simulink model "ITMBS_square_M2"  (R2023a)
settings: Solver=FixedStepDiscrete  StartTime=0.0  StopTime=10.0  FixedStep=0.05  RelTol=1e-3  EnableMultiTasking=on
values from neighbouring files (symbols this model uses):
  dist = 100    [M2_square.m]
libraries: legoev3lib x4
settings Model: ExtModeTrigDuration=2  Creator=3w09  LastModifiedBy=Sachin K S
settings SolverCC: PositivePriorityOrder=on  AutoInsertRateTranBlk=on
settings OptimizationCC: EnhancedBackFolding=on  PassReuseOutputArgsAs=Individual arguments  ZeroExternalMemoryAtStartup=off  ZeroInternalMemoryAtStartup=off  MaxStackSize=64  OptimizeBlockOrder=speed  DifferentSizesBufferReuse=on  OptimizationCustomize=off  EfficientTunableParamExpr=on
settings DebuggingCC: ParameterTunabilityLossMsg=error
settings HardwareCC: ProdBitPerPointer=32  ProdBitPerSizeT=32  ProdBitPerPtrDiffT=32  ProdLargestAtomicInteger=Long  ProdWordSize=32  ProdHWDeviceType=ARM Compatible->ARM 9  UseEmbeddedCoderFeatures=off  UseSimulinkCoderFeatures=off
settings SFSimCC: MATLABDynamicMemAlloc=off
settings RTWCC: Description=Embedded Coder  SystemTargetFile=ert.tlc  HardwareBoard=LEGO MINDSTORMS EV3  TLCOptions="-aInlineSetEventsForThisBaseRateFcn=TLC_FALSE -aSuppressMultiTaskScheduler=TLC_FALSE  -aRateBasedStepFcn=0"  TemplateMakefile=ert_default_tmf  Toolchain=Sourcery G++ Lite v2009q3
settings CodeAppCC: ForceParamTrailComments=on  IgnoreCustomStorageClasses=off  OperatorAnnotations=on  SimulinkDataObjDesc=on  SFDataObjDesc=on  InsertBlockDesc=on
settings ERTTargetCC: SupportContinuousTime=on  SupportNonInlinedSFcns=on  SupportVariableSizeSignals=on  ExtModeTransport=2  ExtModeStaticAlloc=on  ExtModeMexFile=ext_xcp  ExtModeIntrfLevel=Level2 - Open

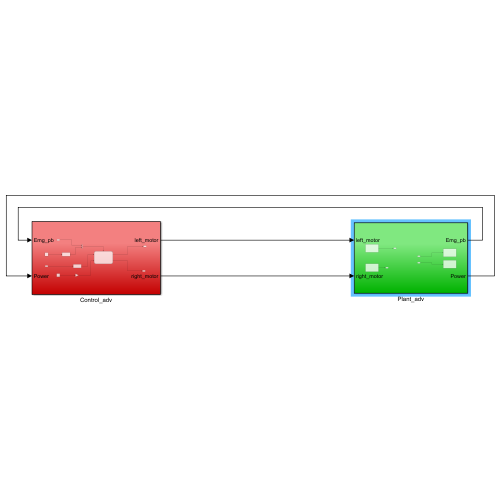
[thumbnail: Simulink's stored preview of the top-level diagram]
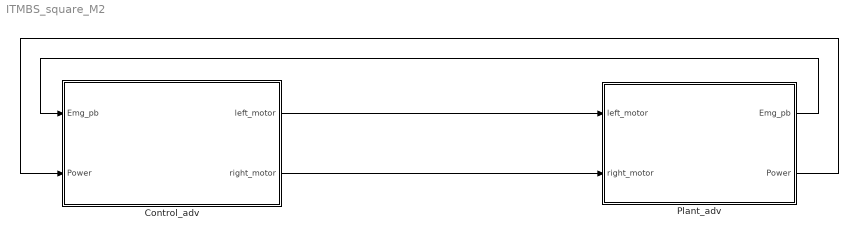
== system ITMBS_square_M2 ==
  Control_adv : Subsystem
  Plant_adv : Subsystem
  wires:
  Plant_adv/1(Emg_pb) -> Control_adv/1(Emg_pb)
  Plant_adv/2(Power) -> Control_adv/2(Power)
  Control_adv/1(left_motor) -> Plant_adv/1(left_motor)
  Control_adv/2(right_motor) -> Plant_adv/2(right_motor)

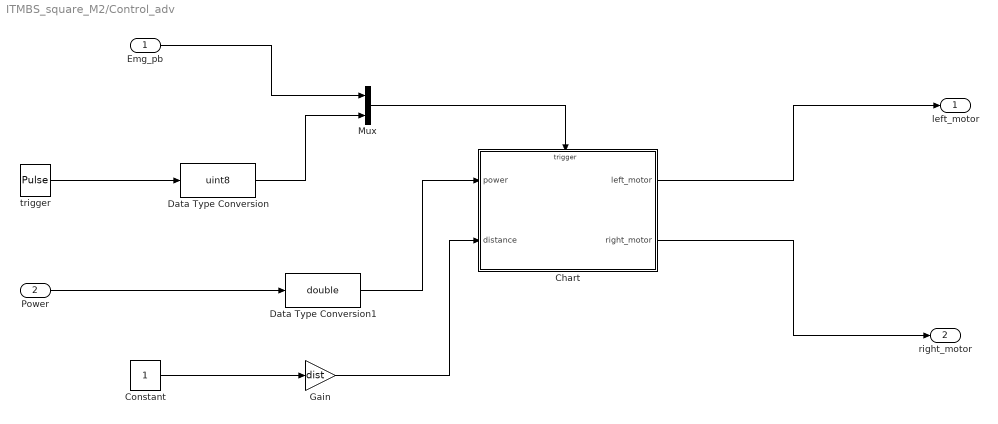
== system ITMBS_square_M2/Control_adv ==
  Emg_pb : Inport
  Power : Inport  Port=2
  Chart : Stateflow chart  TreatAsAtomicUnit=on
  Constant : Constant
  Data Type Conversion : DataTypeConversion  OutDataTypeStr=uint8  SaturateOnIntegerOverflow=off  RndMeth=Floor
  Data Type Conversion1 : DataTypeConversion  OutDataTypeStr=double  SaturateOnIntegerOverflow=off  RndMeth=Floor
  Gain : Gain  Gain=dist
  Mux : Mux  Inputs=2
  trigger : DiscretePulseGenerator  Period=3  PulseWidth=2  SampleTime=0.05
  left_motor : Outport
  right_motor : Outport  Port=2
  wires:
  Constant/1 -> Gain/1
  Emg_pb/1 -> Mux/1
  Chart/2(right_motor) -> right_motor/1
  Gain/1 -> Chart/2(distance)
  Data Type Conversion/1 -> Mux/2
  trigger/1 -> Data Type Conversion/1
  Power/1 -> Data Type Conversion1/1
  Data Type Conversion1/1 -> Chart/1(power)
  Mux/1 -> Chart/Trigger
  Chart/1(left_motor) -> left_motor/1

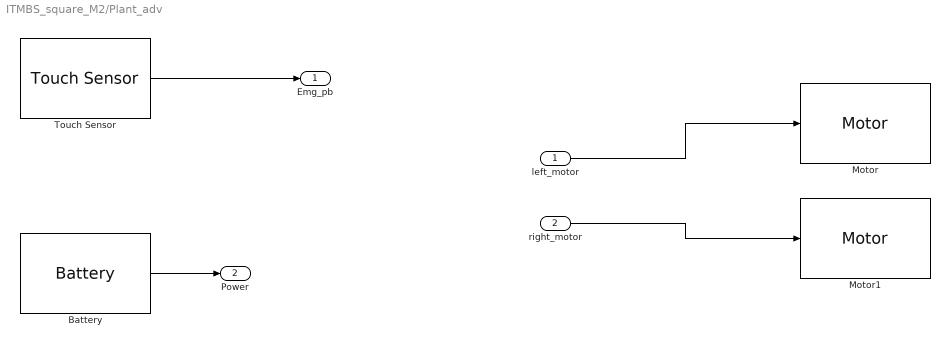
== system ITMBS_square_M2/Plant_adv ==
  left_motor : Inport
  right_motor : Inport  Port=2
  Battery : legoev3lib/Battery  SampleTime=0.1
  Motor : legoev3lib/Motor  sportNumber=A  sstopAction=Brake
  Motor1 : legoev3lib/Motor  sportNumber=B  sstopAction=Brake
  Touch Sensor : legoev3lib/Touch Sensor  portNumber=1  sampleTime=0.1
  Emg_pb : Outport
  Power : Outport  Port=2
  wires:
  Battery/1 -> Power/1
  right_motor/1 -> Motor1/1
  Touch Sensor/1 -> Emg_pb/1
  left_motor/1 -> Motor/1

== stateflow chart ITMBS_square_M2/Control_adv/Chart ==
  settings: executeAtInitialization=1
  state OFF
    entry:
    right_motor=0;
    left_motor=0;
    c=0;
  state ON
    right_motor =power;
    left_motor =power;
  state square
    entry:
    right_motor= 0;
    left_motor=power;
  (default) -> ON
  ON -> OFF [order 1] : [pushbutton_event_input]
  square -> ON [order 2] : [after(0.32,sec)]
  OFF -> (junction 36)
  square -> OFF [order 1] : [pushbutton_event_input]
  ON -> square [order 2] : [after(0.0192* distance ,sec)]
  (junction 38) -> ON [order 1] : [c==2]
  (junction 36) -> (junction 37) [order 1] : [pushbutton_event_input]
  (junction 36) -> (junction 38) [order 2]
  (junction 37) -> (junction 39) : {c= c+1;}
  (junction 39) -> (junction 38)
  (junction 38) -> (junction 53) [order 2]
  data: power input; c local; left_motor output; right_motor output; distance input
  events: pushbutton_event_input input RISING_EDGE_EVENT; trigger input RISING_EDGE_EVENT
